simulink model "fir_example_mb"  (Simulink 7.4)
settings: Solver=VariableStepDiscrete  StartTime=0.0  StopTime=inf  MaxStep=0.2  RelTol=1e-3
undefined symbols (not defined in the file): xlipgetpartsetting
libraries: xbsIndex_r4 x13, xbsCopyrightNotice_r4 x1
settings Model: Creator=jou  LastModifiedBy=jou
settings DebuggingCC: SolverPrmCheckMsg=none

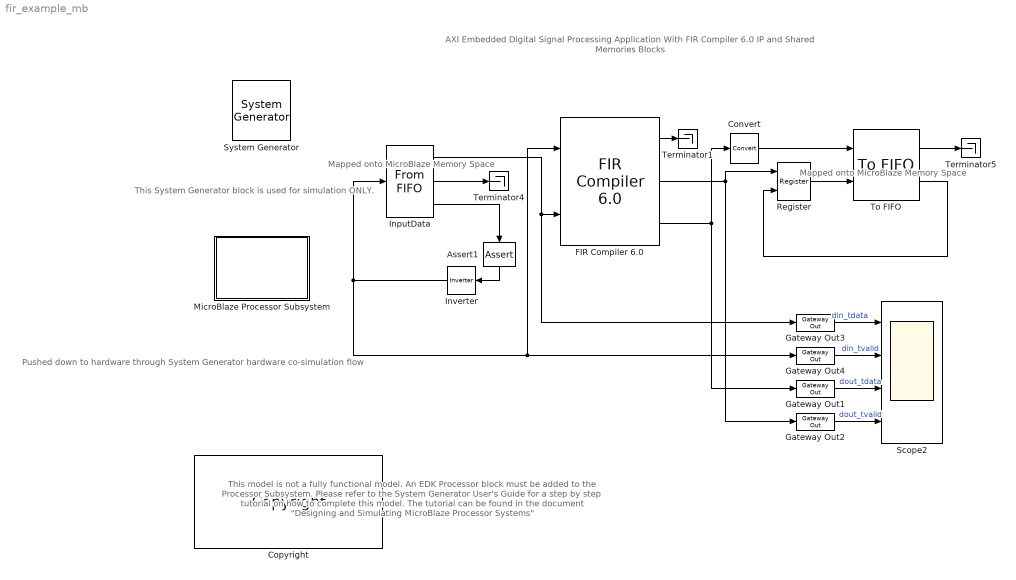
== system fir_example_mb ==
  note: Mapped onto
      | MicroBlaze Memory
      | Space
  note: Mapped onto
      | MicroBlaze Memory
      | Space
  note: AXI Embedded Digital Signal Processing Application With
      | FIR Compiler 6.0 IP and Shared Memories Blocks
  note: Pushed down to hardware through
      | System Generator
      | hardware co-simulation flow
  note: This model is not a fully functional model. An EDK Processor block must
      | be added to the  Processor Subsystem.
      |
      | Please refer to the System Generator User's Guide for a step by step
      | tutorial on how to complete this model. The tutorial can be found
      | in the document "Designing and Simulating MicroBlaze Processor Systems"
  note: This System Generator block is
      | used for simulation ONLY.
  " System Generator" : xbsIndex_r4/ System Generator  Tag=genX  SystemSampleTime=-1  xilinxfamily=spartan6  part=xc6slx16  speed=-2  package=csg324  synthesis_tool=XST  clock_wrapper=Clock Enables  directory=./netlist  testbench=off  simulink_period=1  sysclk_period=20  dcm_input_clock_period=100  incr_netlist=off  trim_vbits=Everywhere in SubSystem  dbl_ovrd=According to Block Masks  core_generation=According to Block Masks  run_coregen=off  deprecated_control=off  eval_field=0  block_type=sysgen
      settings: block_version=8.2.RC1
  Assert1 : xbsIndex_r4/Assert  assert_type=off  type_source=Explicitly  arith_type="Signed  (2's comp)"  n_bits=16  bin_pt=14  assert_rate=on  rate_source=Explicitly  period=1  output_port=on  block_type=assert
      settings: block_version=12.1
  Convert : xbsIndex_r4/Convert  arith_type=Unsigned  n_bits=32  bin_pt=0  quantization=Truncate  overflow=Wrap  en=off  latency=0  dbl_ovrd=off  pipeline=off  block_type=convert
      settings: block_version=12.1
  Copyright : xbsCopyrightNotice_r4/Copyright  copyrighttext="Copyright (c) 2010  by  Xilinx, Inc. All rights reserved.<br><br>This file contains proprietary, confidential information of Xilinx, Inc., is distributed under licensefrom Xilinx, Inc., and may be used, copied and/or disclosed only pursuant to the terms of a valid licenseagreement with Xilinx, Inc. Xilinx hereby grants you a license to use this file solely for design,simulation, implementation and creation of design files limited to Xilinx devices or technologies. Use with non-Xilinx devices or technologies is expressly prohibited and immediately terminates your license unless covered by a separate agreement.<br><br>Xilinx is providing this design, code, or information \"as-is\" solely for use in developing programs and solutions for Xilinx devices, with no obligation on the part of Xilinx to provide support. By providingthis design, code, or information as one possible implementation of this feature, application or standard,Xilinx is making no representation that this implementation is free from any claims of infringement. Youare responsible for obtaining any rights you may require for your implementation. Xilinx expressly disclaimsany warranty whatsoever with respect to the adequacy of the implementation, including but not limited to anywarranties or representations that this implementation is free from claims of infringement, implied warrantiesof merchantability or fitness for a particular purpose.<br><br>Xilinx products are not intended for use in life support appliances, devices, or systems. Use in such applications is expressly prohibited.<br><br>Any modifications that are made to the Source Code are done at the user's sole risk and will be unsupported.<br><br>This copyright and support notice must be retained as part of this text at all times. (c) Copyright 1995-2010 Xilinx, Inc. All rights reserved."  block_type=copyright
      settings: block_version=10.1.00
      settings: infoedit=|
      | Copyright(C) 2007 by  Xilinx, Inc. All rights reserved.<br>
      | <br>
      | This file contains proprietary, confidential information of Xilinx, Inc., is distributed under license
      | from Xilinx, Inc., and may be used, copied and/or disclosed only pursuant to the terms of a valid license
      | agreement with Xilinx, Inc. Xilinx hereby grants you a license to use this file solely for design,
      | simulation, implementation and creation of design files limited to Xilinx devices or technologies. Use
      | with non-Xilinx devices or technologies is expressly prohibited and immediately terminates your license
      | unless covered by a separate agreement.<br>
      | <br>
      | Xilinx is providing this design, code, or information "as-is" solely for use in developing programs and
      | solutions for Xilinx devices, with no obligation on the part of Xilinx to provide support. By providing
      | this design, code, or information as one possible implementation of this feature, application or standard,
      | Xilinx is making no representation that this implementation is free from any claims of infringement. You
      | are responsible for obtaining any rights you may require for your implementation. Xilinx expressly disclaims
      | any warranty whatsoever with respect to the adequacy of the implementation, including but not limited to any
      | warranties or representations that this implementation is free from claims of infringement, implied warranties
      | of merchantability or fitness for a particular purpose.<br>
      | <br>
      | Xilinx products are not intended for use in life support appliances, devices, or systems. Use in such
      | applications is expressly prohibited.<br>
      | <br>
      | Any modifications that are made to the Source Code are done at the user's sole risk and will be unsupported.<br>
      | <br>
      | This copyright and support notice must be retained as part of this text at all times.
      | (c) Copyright 1995-2007 Xilinx, Inc. All rights reserved.
  FIR Compiler 6.0 : xbsIndex_r4/FIR Compiler 6.0   coefficientvector=[1, 2:16]  coefficient_sets=1  filter_type=Single_Rate  interpolation_rate=1  decimation_rate=1  number_channels=1  ratespecification=Sample_Period  sampleperiod=1  hardwareoversamplingrate=1  coefficient_reload=off  coefficient_sign=Unsigned  quantization=Quantize_Only  coefficient_width=18  bestprecision=off  coefficient_fractional_bits=0  coefficient_structure=Inferred  number_paths=1  output_rounding_mode=Full_Precision  output_width=37  optimization_goal=Area  data_buffer_type=Automatic  coefficient_buffer_type=Automatic  input_buffer_type=Automatic  output_buffer_type=Automatic  preference_for_other_storage=Automatic  multi_column_support=Disabled  columnconfig='16'  inter_column_pipe_length=4  data_has_tlast=Not_Required  m_data_has_tready=off  s_data_has_tuser=Not_Required  m_data_has_tuser=Not_Required  s_config_sync_mode=On_Vector  s_config_method=Single  num_reload_slots=1  has_aclken=off  has_aresetn=off  trim_axipin_name=on  passband_min=0.0  passband_max=0.5  stopband_min=0.5  stopband_max=1.0  filter_selection=1  gui_behaviour=Sysgen_GUI  data_sign=Signed  data_width=16  wrapper_available=true  ip_wrap_arbitrary_binary_point=true  ip_name=FIR Compiler  ip_version=6.0  dsptool_ready=true  ipcore_usecache=true  ipcore_useipmodelcache=true  ipcore_xco_need_fpga_part=true  port_translation_map={ 'aclken' => 'en', 'aresetn' => 'rst' }  run_core_at_system_period=true  ipcore_fpga_part=xlipgetpartsetting(gcb, {'virtex6', 'xc6vlx75t', '-3', 'ff784'})  structural_sim=false  block_type=fir_compiler_v6_0
      settings: infoedit=Maximum Possible : Maximizes oversampling rate. Abtracted input handshake (no s_data_tvalid) and automatic rate propagation.<br><br>Hardware Oversampling Rate : Specifies oversampling rate relative to the input sample period. Abtracted input handshake (no s_data_tvalid) and automatic rate propagation.<br><br>Sample Period : Specifies absolute oversampling rate. No input handshake abstraction (exposes s_data_tvalid) and no rate propagation.  block_version=12.3
  Gateway Out{1..4} (4 alike) : xbsIndex_r4/Gateway Out  hdl_port=off  timing_constraint=None  locs_specified=off  LOCs={}  block_type=gatewayout
      settings: infoedit="Gateway out block.  Converts Xilinx fixed point inputs into ouputs of type Simulink integer, double, or fixed point.<br><br>Hardware notes:  In hardware these blocks become top level output ports or are discarded, depending on how they are configured."  block_version=12.1
  InputData : xbsIndex_r4/From FIFO  shared_memory_name='din'  ownership=Owned elsewhere  depth=64  percent_nbits=4  has_arst=off  arith_type=Unsigned  n_bits=32  bin_pt=0  dbl_ovrd=off  mem_type=Block RAM  block_type=fromfifo
      settings: AttributesFormatString=FIFO\n<< %<shared_memory_name> >>  infoedit=First-in-first-out (FIFO) block that reads FIFO data from shared memory storage.  block_version=8.2.RC1
  Inverter : xbsIndex_r4/Inverter  en=off  latency=0  dbl_ovrd=off  block_type=inv
      settings: block_version=12.1
  MicroBlaze Processor Subsystem : Subsystem
  Register : xbsIndex_r4/Register  init=0  rst=on  en=off  dbl_ovrd=off  block_type=register
      settings: block_version=12.0
  Scope2 : Scope  NumInputPorts=4
      settings: TimeRange=600  YMin=0~0~0~0  YMax=1~1~17.5~1
  Terminator1 : Terminator
  Terminator4 : Terminator
  Terminator5 : Terminator
  To FIFO : xbsIndex_r4/To FIFO  shared_memory_name='dout'  ownership=Owned elsewhere  depth=16  percent_nbits=4  has_arst=off  explicit_data_type=on  arith_type=Unsigned  n_bits=32  bin_pt=0  dbl_ovrd=off  mem_type=Block RAM  block_type=tofifo
      settings: AttributesFormatString=FIFO\n<< %<shared_memory_name> >>  infoedit=First-in-first-out (FIFO) block that writes FIFO data to shared memory storage.  block_version=8.2.RC1
  wires:
  To FIFO/1 -> Terminator5/1
  InputData/1 -> Gateway Out3/1, FIR Compiler 6.0/2
  InputData/3 -> Assert1/1
  Inverter/1 -> InputData/1, Gateway Out4/1, FIR Compiler 6.0/1
  InputData/2 -> Terminator4/1
  Assert1/1 -> Inverter/1
  Convert/1 -> To FIFO/1
  Gateway Out3/1 -> Scope2/1  "din_tdata"
  Gateway Out4/1 -> Scope2/2  "din_tvalid"
  Gateway Out1/1 -> Scope2/3  "dout_tdata"
  Gateway Out2/1 -> Scope2/4  "dout_tvalid"
  Register/1 -> To FIFO/2
  To FIFO/2 -> Register/2
  FIR Compiler 6.0/2 -> Register/1, Gateway Out2/1
  FIR Compiler 6.0/1 -> Terminator1/1
  FIR Compiler 6.0/3 -> Convert/1, Gateway Out1/1

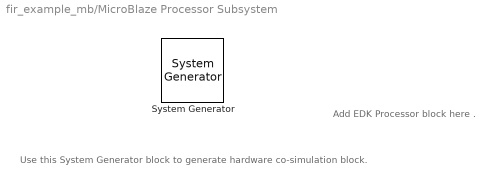
== system fir_example_mb/MicroBlaze Processor Subsystem ==
  note: Add EDK Processor block here
      |
      |
      |
      | .
  note: Use this System Generator block
      | to generate
      | hardware co-simulation block.
  " System Generator" : xbsIndex_r4/ System Generator  Tag=genX  SystemSampleTime=-1  xilinxfamily=spartan6  part=xc6slx16  speed=-2  package=csg324  synthesis_tool=XST  clock_wrapper=Clock Enables  directory=./netlist_sp601_jtag  testbench=off  simulink_period=1  sysclk_period=20  dcm_input_clock_period=100  incr_netlist=off  trim_vbits=Everywhere in SubSystem  dbl_ovrd=According to Block Masks  core_generation=According to Block Masks  run_coregen=off  deprecated_control=off  eval_field=0  block_type=sysgen
      settings: block_version=8.2.RC1
